simulink model "Exercitiul6"  (R2016a)
settings: Solver=VariableStepDiscrete  StartTime=0.0  StopTime=960  RelTol=1e-3
undefined symbols (not defined in the file): m, n
settings Model: Creator=Cristina  LastModifiedBy=Cristina

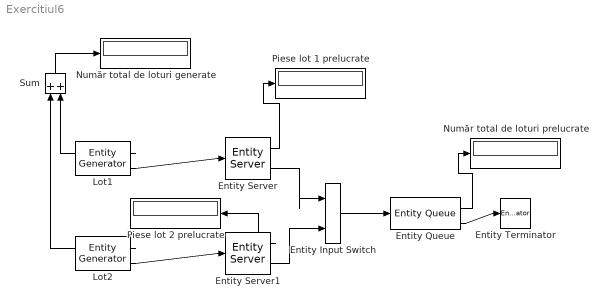
== system Exercitiul6 ==
  Entity Input Switch : EntityInputSwitch  InputPortMessageModes=m,m  OutputPortMessageModes=m
  Entity Queue : EntityQueue  InputPortMessageModes=m  OutputPortMessageModes=n,m  Capacity=inf  NumberEntitiesDeparted=on
      settings: OutputPortMap=o0,o5
  Entity Server : EntityServer  InputPortMessageModes=m  OutputPortMessageModes=n,m  Capacity=1  ServiceTimeSource=MATLAB action  ServiceTimeAction=|  NumberEntitiesDeparted=on
      | persistent init
      | if isempty(init)
      |     rng(125);
      |     init = true;
      | end
      | dt = 14 + 8 * rand;
      settings: OutputPortMap=o0,o9
  Entity Server1 : EntityServer  InputPortMessageModes=m  OutputPortMessageModes=n,m  Capacity=1  ServiceTimeSource=MATLAB action  ServiceTimeAction=|  NumberEntitiesDeparted=on
      | persistent init
      | if isempty(init)
      |     rng(126);
      |     init = true;
      | end
      | dt = 14 + 8 * rand;
      settings: OutputPortMap=o0,o9
  Entity Terminator : EntityTerminator  InputPortMessageModes=m
  Lot1 : EntityGenerator  OutputPortMessageModes=n,m  TimeSource=MATLAB action  IntergenerationTimeAction=|  NumberEntitiesDeparted=on  EntityType=Structured  EntityTypeName=Entity
      | persistent init
      | if isempty(init)
      |     rng(123);
      |     init = true;
      | end
      | dt = 25 + 10 * rand;
      settings: OutputPortMap=o0,o3
  Lot2 : EntityGenerator  OutputPortMessageModes=n,m  TimeSource=MATLAB action  IntergenerationTimeAction=|  NumberEntitiesDeparted=on  EntityType=Structured  EntityTypeName=Entity
      | persistent init
      | if isempty(init)
      |     rng(124);
      |     init = true;
      | end
      | dt = 38 + 14 * rand;
      settings: OutputPortMap=o0,o3
  Număr total de loturi generate : Display
  Număr total de loturi prelucrate : Display
      settings: InputPortMessageModes=m
  Piese lot 1 prelucrate : Display
  Piese lot 2 prelucrate : Display
  Sum : Sum  Inputs=|++
  wires:
  Lot1/2 -> Entity Server/1
  Lot2/2 -> Entity Server1/1
  Entity Input Switch/1 -> Entity Queue/1
  Entity Server/2 -> Entity Input Switch/1
  Entity Server1/2 -> Entity Input Switch/2
  Lot1/1 -> Sum/2
  Lot2/1 -> Sum/1
  Sum/1 -> Număr total de loturi generate/1
  Entity Server/1 -> Piese lot 1 prelucrate/1
  Entity Server1/1 -> Piese lot 2 prelucrate/1
  Entity Queue/1 -> Număr total de loturi prelucrate/1
  Entity Queue/2 -> Entity Terminator/1
